simulink model "Project6"  (R2024b)
settings: Solver=VariableStepAuto  StartTime=0.0  StopTime=10.0  RelTol=1e-3
undefined symbols (not defined in the file): Kd, Ki, Kp
settings Model: Creator=szala  LastModifiedBy=szala

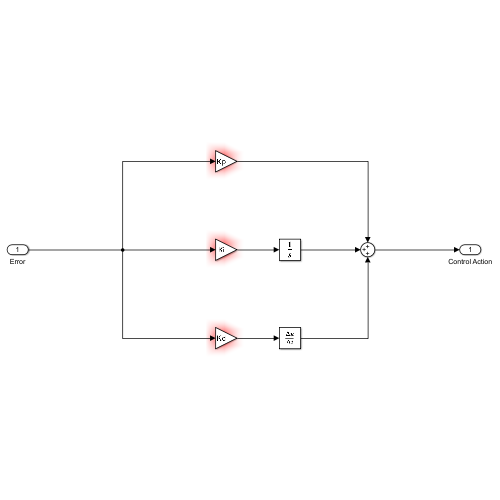
[thumbnail: Simulink's stored preview of the top-level diagram]
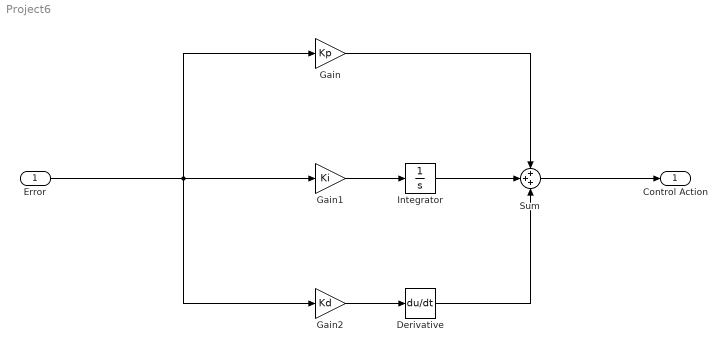
== system Project6 ==
  Error : Inport
  Derivative : Derivative
  Gain : Gain  Gain=Kp
  Gain1 : Gain  Gain=Ki
  Gain2 : Gain  Gain=Kd
  Integrator : Integrator
  Sum : Sum  Inputs=+++
  Control Action : Outport
  wires:
  Error/1 -> Gain/1, Gain1/1, Gain2/1
  Sum/1 -> Control Action/1
  Gain/1 -> Sum/1
  Integrator/1 -> Sum/2
  Gain2/1 -> Derivative/1
  Gain1/1 -> Integrator/1
  Derivative/1 -> Sum/3
